simulink model "balancerPretty"  (Simulink 8.4)
settings: Solver=ode45  StartTime=0.0  StopTime=10.0  RelTol=1e-3
PreLoadFcn:
  | g = 9.8;
  | mp = 1;
  | mw = 0.4e-1;
  | l = .5;
  | r = 0.9e-1;
  | K=[-0.057735026918936,-0.092489763994034,-9.203770713722140,-2.171112972218308];
  | A=[0 1 0 0;0 0 -mp*g/(r*(mp+4*mw)) 0;0 0 0 1;0 0 g*(mp+2*mw)/(l*(mp+4*mw)) 0];
  | B=[0;2/(r*r*(mp+4*mw)); 0; -1/(l*r*(mp+4*mw))];
  | Q=[1 0 0 0;0 1 0 0;0 0 1 0;0 0 0 1]
  | R=1
  | initial=[0.4;0;pi/5;0];
StopFcn:
  | maxdist=max(yout(:,1))*r+r;
  | mindist=min(yout(:,1))*r-r;
  | figure('name','Animation');
  | for i = 1:size(yout,1)
  |     wheelAngle=yout(i,1);
  |     pendulumAngle=-yout(i,3)+pi/2;
  |     axisPoint=[wheelAngle*r 0];
  |     %draw pendulum
  |     plot([axisPoint(1) axisPoint(1)+l*cos(pendulumAngle)],[axisPoint(2) axisPoint(2)+l*sin(pendulumAngle)],'LineWidth',4);
  |     hold on
  |     %draw wheel
  |     th=0:pi/50:2*pi;
  |     xu=r*cos(th)+axisPoint(1);
  |     yu=r*sin(th)+axisPoint(2);
  |     plot(xu,yu,'LineWidth',2);
  | 
  |     plot([axisPoint(1)-r*cos(-wheelAngle) axisPoint(1)+r*cos(-wheelAngle)],[axisPoint(2)-r*sin(-wheelAngle) axisPoint(2)+r*sin(-wheelAngle)],'LineWidth',2);
  |     plot([axisPoint(1)-r*cos(pi/2-wheelAngle) axisPoint(1)+r*cos(pi/2-wheelAngle)],[axisPoint(2)-r*sin(pi/2-wheelAngle) axisPoint(2)+r*sin(pi/2-wheelAngle)],'LineWidth',2);
  |     axis([mindist maxdist mindist maxdist]);
  |     M(i) = getframe;
  |     hold off
  | end
  | movie(M)
libraries: simulink x1
Description:
  | Inverted pendulum on wheel math model with LQR control
  | 
  | Author: Alexander Semion
  | Contacts: spin7ion@gmail.com
  | 
  | Reffer to http://spin7ion.ru/ru/blog/balancerBuildSteps
  | 
  | Variables in workspace:
  | r - Radius of wheel
  | l - Length of pendulum
  | mw - Mass of wheel
  | mp - Mass of pendulum
  | K - LQR coefficients
settings Model: Creator=spin  LastModifiedBy=spin7ion
settings DataIOCC: LimitDataPoints=off  SignalLoggingSaveFormat=Dataset
settings OptimizationCC: ExpressionDepthLimit=128
settings DebuggingCC: UnderspecifiedInitializationDetection=Simplified  MergeDetectMultiDrivingBlocksExec=error  SolverPrmCheckMsg=none  FcnCallInpInsideContextMsg=EnableAllAsError  StateNameClashWarn=none
settings GRTTargetCC: CombineOutputUpdateFcns=on  GRTInterface=off

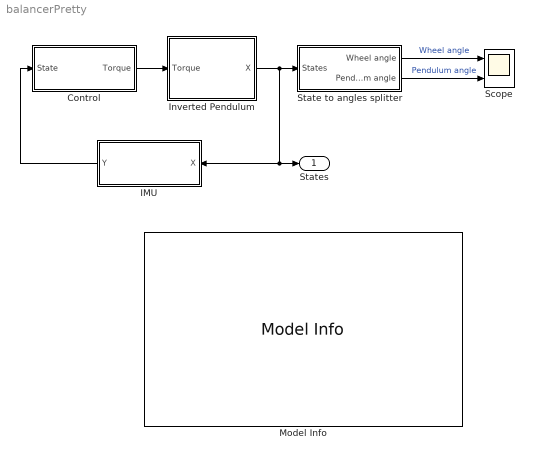
== system balancerPretty ==
  Control : Subsystem
  IMU : Subsystem
  Inverted Pendulum : Subsystem
  Model Info : simulink/Model-Wide Utilities/Model Info  Frame=on  DisplayStringWithTags=|  HorizontalTextAlignment=Center  LeftAlignmentValue=0.5  SourceBlockDiagram=balancerPretty  TagMaxNumber=20
      | %<Description>
      | 
      | %<ModifiedDate>
  Scope : Scope  NumInputPorts=2
      settings: YMin=-8e+11~1.57  YMax=-5e+11~1.5715
  State to angles splitter : Subsystem
  States : Outport
  wires:
  Inverted Pendulum/1(X) -> States/1, IMU/1(X), State to angles splitter/1(States)
  Control/1(Torque) -> Inverted Pendulum/1(Torque)
  IMU/1(Y) -> Control/1(State)
  State to angles splitter/1(Wheel angle) -> Scope/1  "Wheel angle"
  State to angles splitter/2(Pendulum angle) -> Scope/2  "Pendulum angle"

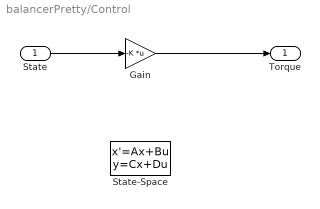
== system balancerPretty/Control ==
  State : Inport
  Gain : Gain  Gain=-K  Multiplication=Matrix(K*u) (u vector)
  State-Space : StateSpace  A=A  B=B  C=eye(4,4)  D=[0;0;0;0]  X0=0
  Torque : Outport
  wires:
  State/1 -> Gain/1
  Gain/1 -> Torque/1

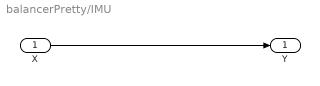
== system balancerPretty/IMU ==
  X : Inport
  Y : Outport
  wires:
  X/1 -> Y/1

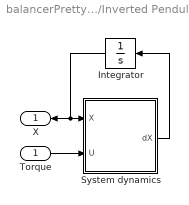
== system balancerPretty/Inverted Pendulum ==
  Torque : Inport  PortDimensions=1
  Integrator : Integrator  InitialCondition=initial
  System dynamics : MATLAB Function  TreatAsAtomicUnit=on
  X : Outport  PortDimensions=4
  wires:
  System dynamics/1(dX) -> Integrator/1
  Torque/1 -> System dynamics/2(U)
  Integrator/1 -> X/1, System dynamics/1(X)

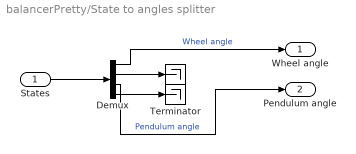
== system balancerPretty/State to angles splitter ==
  States : Inport
  " " : Terminator
  Demux : Demux
  Terminator : Terminator
  Wheel angle : Outport
  Pendulum angle : Outport  Port=2
  wires:
  States/1 -> Demux/1
  Demux/2 -> " "/1
  Demux/4 -> Terminator/1
  Demux/3 -> Pendulum angle/1  "Pendulum angle"
  Demux/1 -> Wheel angle/1  "Wheel angle"

== matlab function Inverted Pendulum/System dynamics ==
  data: X input double size=4; dX output double size=4; U input double; r parameter double size=1; l parameter double size=1; mp parameter double size=1; mw parameter double size=1
function dX = fcn(X,U, r, l, mp, mw)
%#codegen
phi=X(1);
dphi=X(2);
theta=X(3);
dtheta=X(4);
g=9.81;

dX=[
dphi;
(-2*r*sin(theta)*(dtheta)^2*l*mp+cos(theta)*mp*g*sin(theta)*r-2*U)/(r^2*(mp*(cos(theta))^2-2*mp-4*mw));
dtheta;
(cos(theta)*sin(theta)*(dtheta)^2*l*mp*r-g*sin(theta)*r*mp-2*g*sin(theta)*r*mw+cos(theta)*U)/(r*l*(mp*(cos(theta))^2-2*mp-4*mw))
];
